simulink model "problem1"  (R2020b)
settings: Solver=VariableStepAuto  StartTime=0.0  StopTime=10.0  RelTol=1e-3
settings Model: Creator=Nitin  LastModifiedBy=Nitin

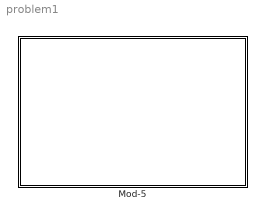
== system problem1 ==
  Mod-5 : Stateflow chart  TreatAsAtomicUnit=on

== stateflow chart problem1/Mod-5 ==
  state state
    [000]
    entry:
    s=0;
    during:
    s=s+1;
    exit:
    s=1;
  state state2
    [010]
    entry:
    s=2;
    during:
    s=s+1;
    exit:
    s=3;
  state state1
    [001]
    entry:
    s=1;
    during:
    s=s+1;
    exit:
    s=2;
  state state4
    [100]
    entry:
    s=4;
    during:
    s=s+1;
    exit:
    s=5;
  state state3
    [011]
    entry:
    s=3;
    during:
    s=s+1;
    exit:
    s=4;
  state1 -> state2 : [s==2]
  state -> state1 : [s==1]
  (default) -> state
  state4 -> state : [s==5]
  state2 -> state3 : [s==3]
  state3 -> state4 : [s==4]
